simulink model "dormand_prince"  (R2023b)
settings: Solver=FixedStepAuto  StartTime=0.0  StopTime=10.0  FixedStep=0.01  RelTol=1e-3
settings Model: Creator=Nacho Andrade  LastModifiedBy=Nacho Andrade

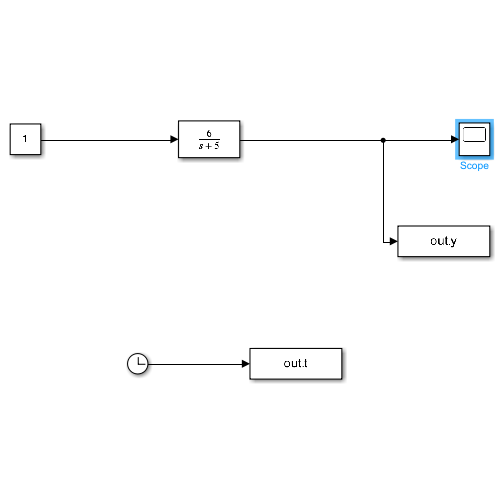
[thumbnail: Simulink's stored preview of the top-level diagram]
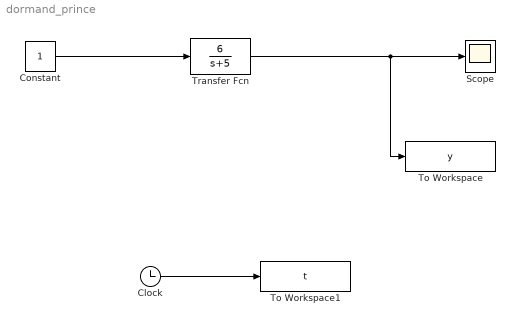
== system dormand_prince ==
  Clock : Clock
  Constant : Constant
  Scope : Scope
  To Workspace : ToWorkspace  VariableName=y  SampleTime=-1
  To Workspace1 : ToWorkspace  VariableName=t  SampleTime=-1
  Transfer Fcn : TransferFcn  Numerator=[6]  Denominator=[1 5]
  wires:
  Clock/1 -> To Workspace1/1
  Transfer Fcn/1 -> To Workspace/1, Scope/1
  Constant/1 -> Transfer Fcn/1
